simulink model "Thyristor_Characterstics_Using_Simulink"  (R2021b)
settings: Solver=VariableStepAuto  StartTime=0.0  StopTime=10.0  RelTol=1e-3
libraries: spsVoltageMeasurementLib x2, spsControlledVoltageSourceLib x1, simulink x1, spsSeriesRLCBranchLib x1, spsThyristorLib x1, spspowerguiLib x1
settings Model: Creator=Vansh  LastModifiedBy=Vansh

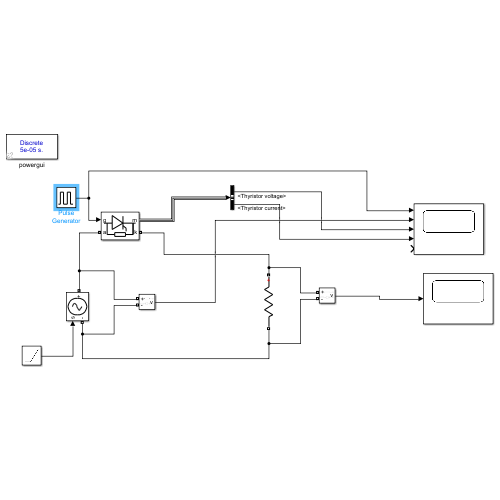
[thumbnail: Simulink's stored preview of the top-level diagram]
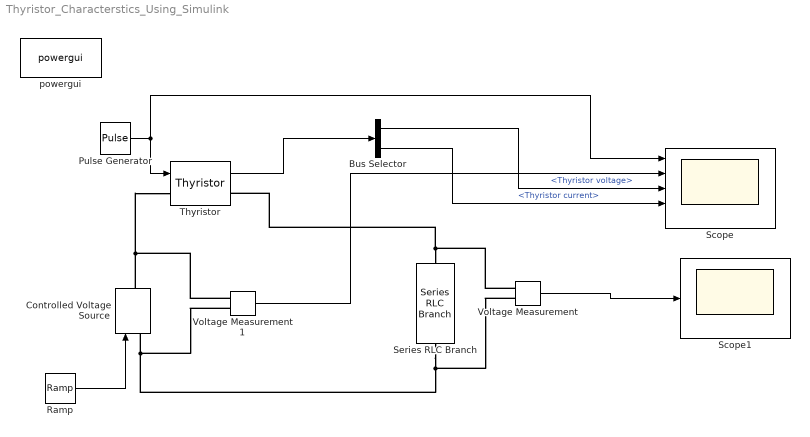
== system Thyristor_Characterstics_Using_Simulink ==
  Bus Selector : BusSelector  OutputSignals=Thyristor voltage,Thyristor current
  Controlled Voltage Source : spsControlledVoltageSourceLib/Controlled Voltage Source  Initialize=on  Source_Type=DC  Amplitude=10  Phase=0  Frequency=0  Measurements=Voltage
  Pulse Generator : DiscretePulseGenerator  PulseType=Time based  Period=4  PulseWidth=5
  Ramp : simulink/Sources/Ramp  slope=1  start=0  InitialOutput=0
  Scope : Scope  NumInputPorts=5
  Scope1 : Scope
  Series RLC Branch : spsSeriesRLCBranchLib/Series RLC Branch  LConnTagsString=__new0  RConnTagsString=__new0  BranchType=R  Resistance=2  Inductance=1e-3  SetiL0=off  InitialCurrent=0  Capacitance=1e-6  Setx0=off  InitialVoltage=0  Measurements=None
  Thyristor : spsThyristorLib/Thyristor  Ron=0.001  Lon=0  Vf=0.8  IC=0  Rs=500  Cs=250e-9  Measurements=on
  Voltage Measurement : spsVoltageMeasurementLib/Voltage Measurement  PhasorSimulation=off  OutputType=Complex  PSBequivalent=0
  Voltage Measurement1 : spsVoltageMeasurementLib/Voltage Measurement  PhasorSimulation=off  OutputType=Complex  PSBequivalent=0
  powergui : spspowerguiLib/powergui  Priority=1  SimulationMode=Discrete  SampleTime=50e-6  frequency=60  Iterations=50  frequencyindice=0  Pbase=100e6  ErrMax=1e-4  UnitsV=kV  UnitsW=MW  buscounter=0  FunctionMessages=off  echomessages=off  EnableUseOfTLC=off  CurrentSourceSwitches=off  DisableSnubberDevices=off  DisableRonSwitches=off  DisableVfSwitches=off  DisplayEquations=off  AutomaticDiscreteSolvers=off  SolverType=Tustin/Backward Euler (TBE)  Interpol=off  ExternalGateDelay=off  methode=off  Ts=100  x0status=blocks  SPID=on  SwTol=0  HookPort=off  NonlinearTolerance=1e-4  nMaxIteration=100  ContinueOnMaxIteration=off  RestoreLinks=warning  ResistiveCurrentMeasurement=off  Frange=[0:2:500]  Ylog=off  Xlog=on  ShowGrid=off  save=off  variable=ZData  structure=0  ZoomFFT=off  StartTime=0.0  cycles=1  DisplayStyle=1  fundamental=60  FreqAxis=off  MaxFrequency=1000  frequencyindicesteady=1  RmsSteady=1  display=off
  wires:
  Bus Selector/1 -> Scope/3  "<Thyristor voltage>"
  Bus Selector/2 -> Scope/4  "<Thyristor current>"
  Pulse Generator/1 -> Thyristor/1, Scope/1
  Thyristor/1 -> Bus Selector/1
  Ramp/1 -> Controlled Voltage Source/1
  Voltage Measurement1/1 -> Scope/2
  Voltage Measurement/1 -> Scope1/1
  connections:
  Controlled Voltage Source/RConn1 -- Thyristor/LConn1 -- Voltage Measurement1/LConn1
  Series RLC Branch/RConn1 -- Voltage Measurement/LConn2 -- Voltage Measurement1/LConn2 -- Controlled Voltage Source/LConn1
  Series RLC Branch/LConn1 -- Thyristor/RConn1 -- Voltage Measurement/LConn1
